simulink model "chap9_5sim"  (Simulink 8.1)
settings: Solver=ode45  StartTime=0.0  StopTime=30  RelTol=1e-3
settings Model: Creator=liujk  LastModifiedBy=liujk
settings DataIOCC: SignalLoggingName=sigsOut
settings OptimizationCC: ExpressionDepthLimit=128
settings DebuggingCC: SaveWithParameterizedLinksMsg=none  SignalResolutionControl=TryResolveAllWithWarning  SolverPrmCheckMsg=none  MultiTaskDSMMsg=warning  MultiTaskCondExecSysMsg=none  StrictBusMsg=None
settings HardwareCC: TargetUnknown=on
settings RTWCC: IncludeERTFirstTime=on

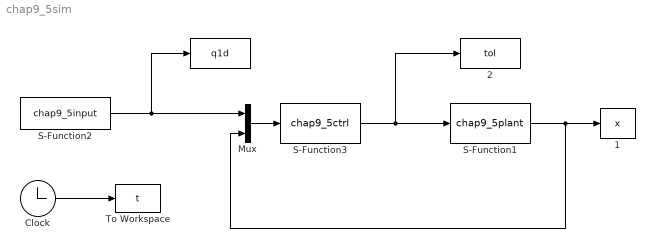
== system chap9_5sim ==
  "  " : ToWorkspace  VariableName=q1d  SampleTime=-1
  "  1" : ToWorkspace  VariableName=x  SampleTime=-1
  "  2" : ToWorkspace  VariableName=tol  SampleTime=-1
  Clock : Clock
  Mux : Mux  Inputs=2
  S-Function1 : S-Function  FunctionName=chap9_5plant  EnableBusSupport=off
  S-Function2 : S-Function  FunctionName=chap9_5input  EnableBusSupport=off
  S-Function3 : S-Function  FunctionName=chap9_5ctrl  EnableBusSupport=off
  To Workspace : ToWorkspace  VariableName=t  SampleTime=-1
  wires:
  Clock/1 -> To Workspace/1
  S-Function2/1 -> Mux/1, "  "/1
  Mux/1 -> S-Function3/1
  S-Function3/1 -> S-Function1/1, "  2"/1
  S-Function1/1 -> "  1"/1, Mux/2
